simulink model "DATA"  (R2018b)
settings: Solver=FixedStepAuto  StartTime=0.0  StopTime=5  FixedStep=0.0005  RelTol=1e-3
settings Model: Creator=User  LastModifiedBy=User

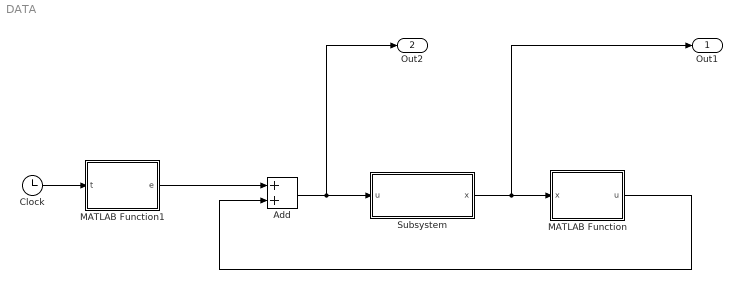
== system DATA ==
  Add : Sum
  Clock : Clock
  MATLAB Function : MATLAB Function  TreatAsAtomicUnit=on
  MATLAB Function1 : MATLAB Function  TreatAsAtomicUnit=on
  Subsystem : Subsystem
  Out1 : Outport
  Out2 : Outport  Port=2
  wires:
  Subsystem/1(x) -> Out1/1, MATLAB Function/1(x)
  MATLAB Function/1(u) -> Add/2
  MATLAB Function1/1(e) -> Add/1
  Clock/1 -> MATLAB Function1/1(t)
  Add/1 -> Out2/1, Subsystem/1(u)

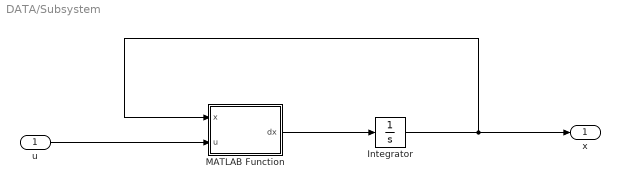
== system DATA/Subsystem ==
  u : Inport
  Integrator : Integrator  InitialCondition=[1;-1]
  MATLAB Function : MATLAB Function  TreatAsAtomicUnit=on
  x : Outport
  wires:
  u/1 -> MATLAB Function/2(u)
  MATLAB Function/1(dx) -> Integrator/1
  Integrator/1 -> MATLAB Function/1(x), x/1

== matlab function DATA/MATLAB Function ==
  data: x input; u output
function u = fcn(x)
x1=x(1);
x2=x(2);
u=-3/2*sin(x1)*(x1+x2);
end

== matlab function DATA/Subsystem/MATLAB Function ==
  data: x input; u input; dx output
function dx = fcn(x,u)
x1=x(1);
x2=x(2);
dx=[-x1+x2;
    -1/2*(x1+x2)+1/2*x2*(1+2*x2^2)*sin(x1)^2+sin(x1)*u];
end

== matlab function DATA/MATLAB Function1 ==
  data: t input; e output
function e = fcn(t)
w=  [-33.7818
   29.4285
  -18.8785
    2.8533
  -33.4351
   10.1982
  -23.7029
   15.4079
   18.9215
   24.8152
   -4.9458
  -41.6179
  -27.1023
   41.3337
  -34.7622
   32.5817
    3.8342
   49.6135
  -42.1824
   -5.7322
  -39.3347
   46.1898
  -49.5366
   27.4910
   31.7303
   36.8695
  -41.5564
  -10.0217
  -24.0130
   30.0068
   -6.8586
   41.0648
  -31.8153
  -23.6197
  -35.4461
  -36.3931
   36.9292
    7.9705
    4.9860
  -35.5045
   35.3031
   12.2055
  -14.9048
    1.3250
   -9.8192
  -42.4033
  -26.0084
  -37.6681
  -31.6092
  -26.0047
   -8.2733
  -45.0346
   40.2716
   44.4787
   -0.9136
   -1.0747
  -16.2281
   40.0054
  -13.0753
  -38.8797
   28.0252
  -11.0261
  -25.8309
   -9.6088
  -40.3545
  -36.8027
   44.2051
   45.6135
    7.5209
  -44.0220
  -26.5220
  -14.6841
   32.1194
  -48.4597
  -45.6976
  -33.1010
   14.9115
   23.1722
   14.7746
   -4.9076
    4.7009
  -20.3679
   24.4693
  -31.1045
   18.6775
  -31.6489
  -13.1515
   12.5619
   28.0227
  -41.8874
   42.9386
   27.5713
   -1.3208
   -6.4141
   -5.3216
  -19.3651
    0.8509
    1.0772
   31.7628
   29.4831];
e=0;
for i=1:100
    e=e+0.005*sin(w(i)*t);
end
end
